simulink model "DigitalInput_model"  (R2016b)
settings: Solver=FixedStepAuto  StartTime=0.0  StopTime=tFinal  FixedStep=T  RelTol=1e-3  EnableMultiTasking=on
values from neighbouring files (symbols this model uses):
  repeatingPulsePeriod = 1    [MAIN_DigitalInput.m]
  repeatingPulseWidthPercent = 30    [MAIN_DigitalInput.m]
libraries: arduinolib x3
settings Model: SimulationMode=external  Creator=Christopher  LastModifiedBy=Christopher
settings DataIOCC: LimitDataPoints=on  StreamToWorkspace=on
settings OptimizationCC: LifeSpan=1  MaxStackSize=64
settings DebuggingCC: AllowSymbolicDim=off  SFUnexpectedBacktrackingDiag=warning  SFNoUnconditionalDefaultTransitionDiag=warning  SFExecutionAtInitializationDiag=none
settings HardwareCC: ProdBitPerPointer=32  ProdBitPerSizeT=32  ProdBitPerPtrDiffT=32  ProdLargestAtomicInteger=Long  ProdLargestAtomicFloat=Double  ProdWordSize=32  ProdHWDeviceType=ARM Compatible->ARM Cortex  UseEmbeddedCoderFeatures=off  UseSimulinkCoderFeatures=off
settings ModelReferenceCC: PropagateSignalLabelsOutOfModel=off
settings RTWCC: SystemTargetFile=ert.tlc  HardwareBoard=Arduino Due  TLCOptions=-aInlineSetEventsForThisBaseRateFcn=TLC_FALSE -aSuppressMultiTaskScheduler=TLC_FALSE -aRateBasedStepFcn=1  TemplateMakefile=ert_default_tmf  Description=Embedded Coder  Toolchain=Arduino ARM v1.6.7  BuildConfiguration=Faster Runs
settings CodeAppCC: IgnoreCustomStorageClasses=off
settings ERTTargetCC: SupportContinuousTime=on  SupportNonInlinedSFcns=on  SupportVariableSizeSignals=on  ConvertIfToSwitch=off  SuppressUnreachableDefaultCases=off
settings ConfigComp: CovMetricSettings=dw  CovHtmlReporting=on  CovSaveCumulativeToWorkspaceVar=on  CovSaveSingleToWorkspaceVar=on  CovExternalEMLEnable=off

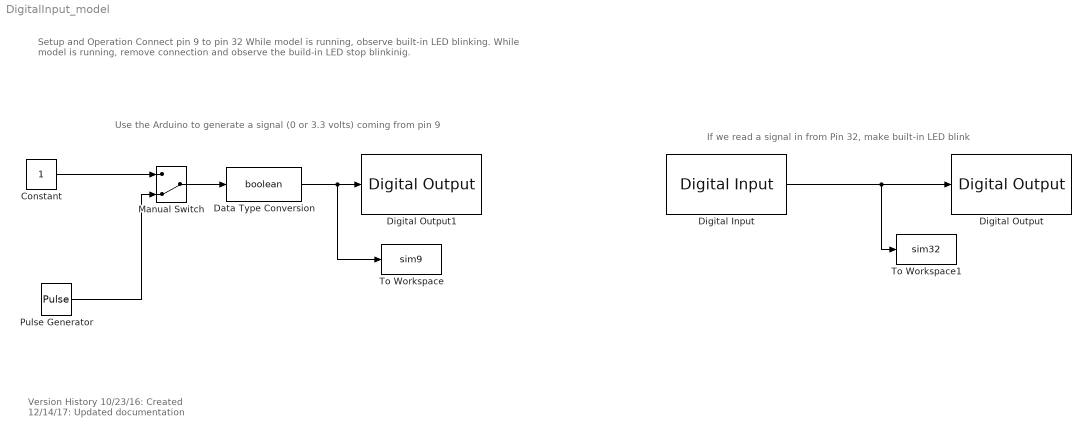
== system DigitalInput_model ==
  note: Setup and Operation
      | Connect pin 9 to pin 32
      | While model is running, observe built-in LED blinking.
      | While model is running, remove connection and observe the build-in LED stop blinkinig.
  note: Version History
      | 10/23/16: Created
      | 12/14/17: Updated documentation
  note: Use the Arduino to generate a signal (0 or 3.3 volts) coming from pin 9
  note: If we read a signal in from Pin 32, make built-in LED blink
  Constant : Constant
  Data Type Conversion : DataTypeConversion  OutDataTypeStr=boolean
  Digital Input : arduinolib/Digital Input  pinNumber=32  sampleTime=T  blockPlatform=arduino
  Digital Output : arduinolib/Digital Output  pinNumber=13  blockPlatform=arduino
  Digital Output1 : arduinolib/Digital Output  pinNumber=9  blockPlatform=arduino
  Manual Switch : ManualSwitch  CurrentSetting=0
  Pulse Generator : DiscretePulseGenerator  PulseType=Time based  Period=repeatingPulsePeriod  PulseWidth=repeatingPulseWidthPercent
  To Workspace : ToWorkspace  VariableName=sim9  SaveFormat=Structure With Time  SampleTime=-1
  To Workspace1 : ToWorkspace  VariableName=sim32  SaveFormat=Structure With Time  SampleTime=-1
  wires:
  Data Type Conversion/1 -> To Workspace/1, Digital Output1/1
  Constant/1 -> Manual Switch/1
  Digital Input/1 -> To Workspace1/1, Digital Output/1
  Manual Switch/1 -> Data Type Conversion/1
  Pulse Generator/1 -> Manual Switch/2
